simulink model "test_behaviour_auto_cst_current_all_v"  (R2022a)
settings: Solver=VariableStepAuto  StartTime=0.0  StopTime=20  RelTol=1e-3
values from neighbouring files (symbols this model uses):
  dfm = dfm_def    (= 0)    [autotest.m]    (also in flCurvesODEModel.m; freqStat.m = fieldOrDefault(params, "dfm", 0.0))
  dsm = values(i)    [autotest.m]    (also in flCurvesODEModel.m = -0.5; freqStat.m = fieldOrDefault(params, "dsm", -0.5))
  dsp = dsp_def    (= 0.5)    [autotest.m]    (also in flCurvesODEModel.m; freqStat.m = fieldOrDefault(params, "dsp", 0.5))
  dup = dup_def    (= -0.5)    [autotest.m]    (also in flCurvesODEModel.m; freqStat.m = fieldOrDefault(params, "dup", -0.5))
  gfm = gfm_def    (= -2)    [autotest.m]    (also in flCurvesODEModel.m; freqStat.m = fieldOrDefault(params, "gfm", -2))
  gsm = gsm_def    (= -4)    [autotest.m]    (also in flCurvesODEModel.m = -2; freqStat.m = fieldOrDefault(params, "gsm", -4))
  gsp = gsp_def    (= 6)    [autotest.m]    (also in flCurvesODEModel.m; freqStat.m = fieldOrDefault(params, "gsp", 6))
  gup = gup_def    (= 5)    [autotest.m]    (also in flCurvesODEModel.m = 0; freqStat.m = fieldOrDefault(params, "gup", 5))
  Iapp = timeseries(Iin,time)    [autotest.m]    (also in flCurvesODEModel.m = @(t) I0; freqStat.m = timeseries(Iapp_val, time); tests.m = -1)
  sampleTime = 0.0001    [autotest.m]    (also in freqStat.m = fieldOrDefault(params, "sampleTime", 0.0001))
undefined symbols (not defined in the file or in its folder): noisePwr
libraries: simulink x1
settings Model: Creator=chris  LastModifiedBy=chris

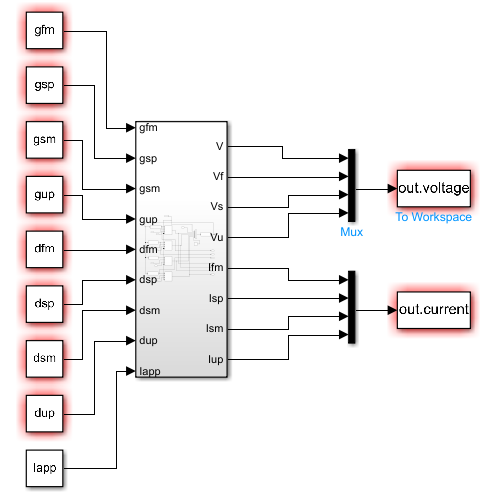
[thumbnail: Simulink's stored preview of the top-level diagram]
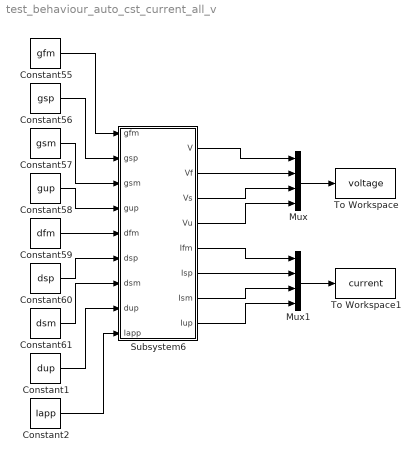
== system test_behaviour_auto_cst_current_all_v ==
  Constant1 : Constant  Value=dup
  Constant2 : Constant  Value=Iapp  LockScale=on
  Constant55 : Constant  Value=gfm
  Constant56 : Constant  Value=gsp
  Constant57 : Constant  Value=gsm
  Constant58 : Constant  Value=gup
  Constant59 : Constant  Value=dfm
  Constant60 : Constant  Value=dsp
  Constant61 : Constant  Value=dsm
  Mux : Mux
  Mux1 : Mux
  Subsystem6 : Subsystem
  To Workspace : ToWorkspace  VariableName=voltage  SaveFormat=Structure With Time  SampleTime=sampleTime
  To Workspace1 : ToWorkspace  VariableName=current  SaveFormat=Structure With Time  SampleTime=sampleTime
  wires:
  Constant56/1 -> Subsystem6/2(gsp)
  Constant58/1 -> Subsystem6/4(gup)
  Constant59/1 -> Subsystem6/5(dfm)
  Constant57/1 -> Subsystem6/3(gsm)
  Constant55/1 -> Subsystem6/1(gfm)
  Constant60/1 -> Subsystem6/6(dsp)
  Constant61/1 -> Subsystem6/7(dsm)
  Constant1/1 -> Subsystem6/8(dup)
  Constant2/1 -> Subsystem6/9(Iapp)
  Mux/1 -> To Workspace/1
  Mux1/1 -> To Workspace1/1
  Subsystem6/1(V) -> Mux/1
  Subsystem6/2(Vf) -> Mux/2
  Subsystem6/3(Vs) -> Mux/3
  Subsystem6/4(Vu) -> Mux/4
  Subsystem6/5(Ifm) -> Mux1/1
  Subsystem6/6(Isp) -> Mux1/2
  Subsystem6/7(Ism) -> Mux1/3
  Subsystem6/8(Iup) -> Mux1/4

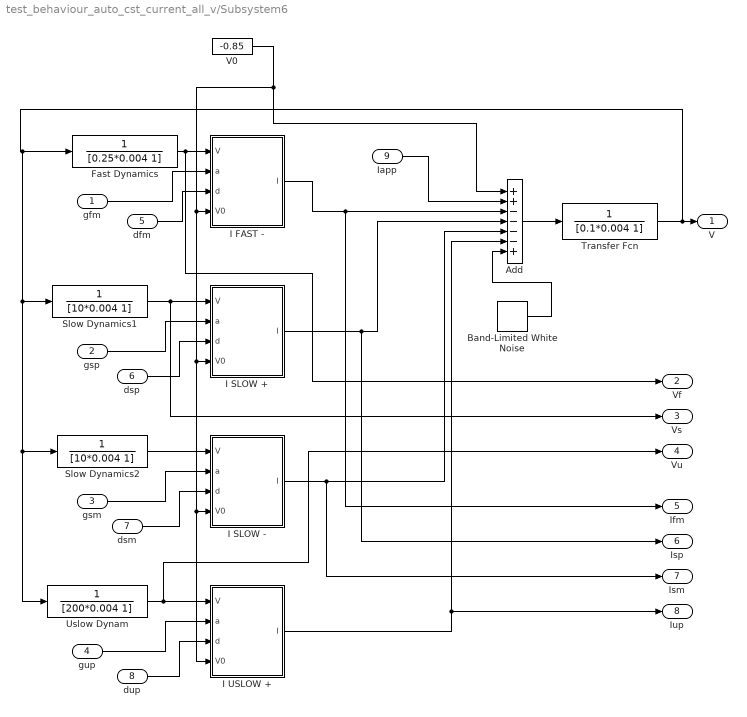
== system test_behaviour_auto_cst_current_all_v/Subsystem6 ==
  gfm : Inport
  gsp : Inport  Port=2
  gsm : Inport  Port=3
  gup : Inport  Port=4
  dfm : Inport  Port=5
  dsp : Inport  Port=6
  dsm : Inport  Port=7
  dup : Inport  Port=8
  Iapp : Inport  Port=9
  Add : Sum  Inputs=++----+
  Band-Limited White Noise : simulink/Sources/Band-Limited White Noise  Cov=[noisePwr]  Ts=0.001  seed=floor(rand(1)*250000)
  Fast Dynamics : TransferFcn  Denominator=[0.25*0.004 1]
  I FAST - : MATLAB Function  TreatAsAtomicUnit=on
  I SLOW + : MATLAB Function  TreatAsAtomicUnit=on
  I SLOW - : MATLAB Function  TreatAsAtomicUnit=on
  I USLOW + : MATLAB Function  TreatAsAtomicUnit=on
  Slow Dynamics1 : TransferFcn  Denominator=[10*0.004 1]
  Slow Dynamics2 : TransferFcn  Denominator=[10*0.004 1]
  Transfer Fcn : TransferFcn  Denominator=[0.1*0.004 1]
  Uslow Dynam : TransferFcn  Denominator=[200*0.004 1]
  V0 : Constant  Value=-0.85
  V : Outport
  Vf : Outport  Port=2
  Vs : Outport  Port=3
  Vu : Outport  Port=4
  Ifm : Outport  Port=5
  Isp : Outport  Port=6
  Ism : Outport  Port=7
  Iup : Outport  Port=8
  wires:
  dup/1 -> I USLOW +/3(d)
  gsm/1 -> I SLOW -/2(a)
  dsm/1 -> I SLOW -/3(d)
  gup/1 -> I USLOW +/2(a)
  Iapp/1 -> Add/2
  Uslow Dynam/1 -> Vu/1, I USLOW +/1(V)
  Add/1 -> Transfer Fcn/1
  Slow Dynamics1/1 -> I SLOW +/1(V), Vs/1
  Slow Dynamics2/1 -> I SLOW -/1(V)
  I FAST -/1(I) -> Add/3, Ifm/1
  I USLOW +/1(I) -> Add/6, Iup/1
  V0/1 -> I USLOW +/4(V0), I SLOW -/4(V0), I SLOW +/4(V0), I FAST -/4(V0), Add/1
  dsp/1 -> I SLOW +/3(d)
  gsp/1 -> I SLOW +/2(a)
  dfm/1 -> I FAST -/3(d)
  gfm/1 -> I FAST -/2(a)
  Fast Dynamics/1 -> I FAST -/1(V), Vf/1
  I SLOW -/1(I) -> Ism/1, Add/5
  Transfer Fcn/1 -> Uslow Dynam/1, Slow Dynamics2/1, Slow Dynamics1/1, Fast Dynamics/1, V/1
  I SLOW +/1(I) -> Isp/1, Add/4
  Band-Limited White Noise/1 -> Add/7

== matlab function test_behaviour_auto_cst_current_all_v/Subsystem6/I FAST - ==
  data: V input; I output; a input; d input; V0 input
function I = fcn(V,a,d,V0)

I = a*(tanh(V-d)-tanh(V0-d));

== matlab function test_behaviour_auto_cst_current_all_v/Subsystem6/I SLOW + ==
  data: V input; I output; a input; d input; V0 input
function I = fcn(V,a,d,V0)

I = a*(tanh(V-d)-tanh(V0-d));

== matlab function test_behaviour_auto_cst_current_all_v/Subsystem6/I SLOW - ==
  data: V input; I output; a input; d input; V0 input
function I = fcn(V,a,d,V0)

I = a*(tanh(V-d)-tanh(V0-d));

== matlab function test_behaviour_auto_cst_current_all_v/Subsystem6/I USLOW + ==
  data: V input; I output; a input; d input; V0 input
function I = fcn(V,a,d,V0)

I = a*(tanh(V-d)-tanh(V0-d));
